simulink library "library_ALICAT_PRESSURE_RW"  (R2024b)
settings: Solver=VariableStepAuto  StartTime=0.0  StopTime=10.0  RelTol=1e-3
undefined symbols (not defined in the file): Controller
settings Model: Creator=GavinWilliamson  LastModifiedBy=GavinWilliamson

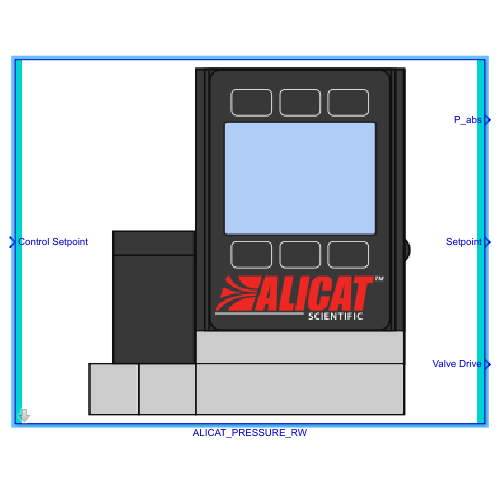
[thumbnail: Simulink's stored preview of the top-level diagram]
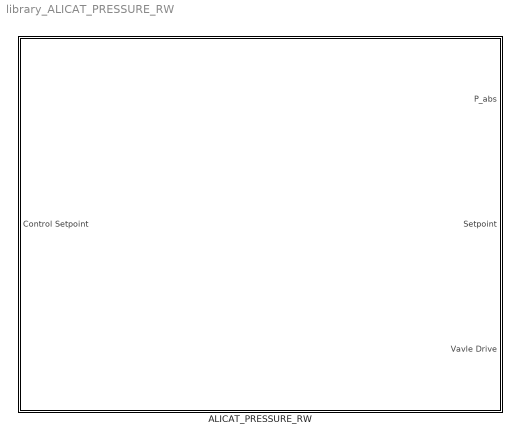
== system library_ALICAT_PRESSURE_RW ==
  ALICAT_PRESSURE_RW : Subsystem  mask{Port="COM4", Device_Name='A', dv_typ=Controller, vlv_typ=on, vlvDR_sw=on, cntrl_sw=on, contrl_typ=Absolute Pressure}
      mask prompts: Device_Name "Device Identifier"; dv_typ "Device Type"; vlv_typ "Two Valve Controller"; vlvDR_sw "Enable Valve Drive Recording"; cntrl_sw "Enable ALICAT Controller"; contrl_typ "Setpoint Variable"
      mask help: Default Mask
      mask Help: web(which('help_ALICAT_PRESSURE_RW.html'), '-helpbrowser')
      mask TypeOptions Port:
      | Level-2 MATLAB
      | S-Function/Port
      mask TypeOptions Device_Name:
      | Level-2 MATLAB
      | S-Function/Device_Name
      mask TypeOptions dv_typ:
      | Level-2 MATLAB
      | S-Function/dv_typ
      mask TypeOptions vlv_typ:
      | Level-2 MATLAB
      | S-Function/vlv_typ
      mask TypeOptions vlvDR_sw:
      | Level-2 MATLAB
      | S-Function/vlvDR_sw
      mask TypeOptions cntrl_sw:
      | Level-2 MATLAB
      | S-Function/cntrl_sw
      mask TypeOptions contrl_typ:
      | Level-2 MATLAB
      | S-Function/contrl_typ
      mask DialogControl Container3 Prompt: General
      mask DialogControl DescGroupVar_copy Prompt: ALICAT_RW
      mask DialogControl DescTextVar_copy Prompt: Block controls and reads an ALICAT pressure device over serial communication. Labels on the ports on the block will disappear if there are not valid for the configuration selected. To see all port labels you can look under the mask of this block.
      mask DialogControl Container10 Prompt: Communication Parameters
      mask DialogControl Container21 Prompt: Device Information
      mask DialogControl Container11 Prompt: Data Logging Options
      mask DialogControl Container12 Prompt: Control Options
      mask DialogControl Container5 Prompt: Instructions
      mask DialogControl Container6 Prompt: Inputs
      mask DialogControl Control2 Prompt: Control Setpoint: The setpoint that you want to write to the device if control mode is enabled. If control mode is disabled this input will no do anything.
      mask DialogControl Container7 Prompt: Register Parameters
      mask DialogControl Container18 Prompt: Communication Parameters
      mask DialogControl Control16 Prompt: Port: Communication port that ALICAT is connected to [string]
      mask DialogControl Control14 Prompt: Device Identifier: Unit ID of ALICAT [char]
      mask DialogControl Container13 Prompt: Device Information
      mask DialogControl Control7 Prompt: Device Type: Select whether the ALICAT that is connected to the COM Port is a controller or meter. This is important to ensure invalid commands are not sent to the device, and to ensure that the outputted data is in the expected format.
      mask DialogControl Control12 Prompt: Two Valve Controller: Select this option if you controller has two control valves
      mask DialogControl Container14 Prompt: Data Logging Options
      mask DialogControl Control8 Prompt: Enable Valve Drive Recording: This will set the valve drive position to be outputted by an ALICAT controller and will also set the value to display on the screen.
      mask DialogControl Container15 Prompt: Control Options
      mask DialogControl Control9 Prompt: Enable ALICAT Controller: This allows an ALICAT controller to be controlled through Simulink. If unchecked, Simulink will just configure the data logging option parameters and read the device outputs.
      mask DialogControl Container16 Prompt: Setpoint Variable
      mask DialogControl Control10 Prompt: If set to "Valve Drive", "Control Setpoint" should be set to the percentage open on the range of 0-100. Where 0 corresponds to closed and 100 corresponds to fully open.  If you have a two valve device the range 0-100 controls the left valve and  0 to -100 controls the right valve.
      mask Display:
      | image('AlicatMFCIcon.png', [0,0,0,0,100,100]);
      | 
      | %input ports
      | if strcmp(get_param(gcb,'cntrl_sw'),'on')
      |     port_label('input', 1, 'Control Setpoint');
      | end
      | 
      | %output ports
      | port_label('output', 1, 'P_abs');
      | if strcmp(get_param(gcb,'dv_typ'),'Controller')
      |     port_label('output', 2, 'Setpoint');
      | end
      | if strcmp(get_param(gcb,'vlvDr_sw'),'on')
      |     port_label('output', 3, 'Valve Drive');
      | end

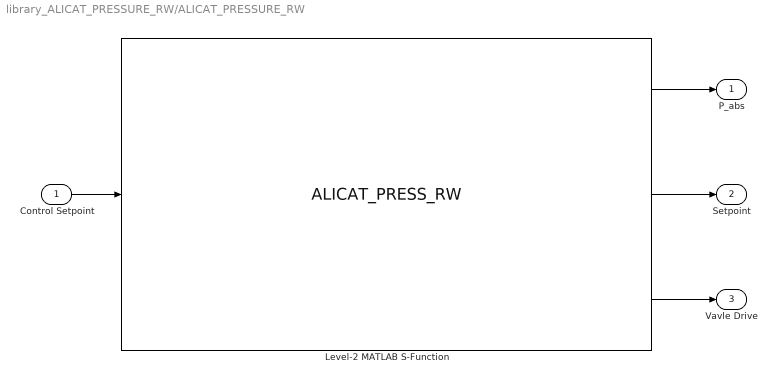
== system library_ALICAT_PRESSURE_RW/ALICAT_PRESSURE_RW ==
  Control Setpoint : Inport
  Level-2 MATLAB S-Function : M-S-Function  FunctionName=ALICAT_PRESS_RW  Parameters=Port, Device_Name, contrl_typ, cntrl_sw, dv_typ,vlvDR_sw,vlv_typ  mask{Port=Port, Device_Name=Device_Name, vlvDR_sw=on, cntrl_sw=on, contrl_typ=Absolute Pressure, dv_typ=Controller, vlv_typ=on}
      mask prompts: Device_Name "Device Identifier"; vlvDR_sw "Enable Valve Drive Recording"; cntrl_sw "Enable ALICAT Controller"; contrl_typ "Setpoint Variable"; dv_typ "Device Type"; vlv_typ "Two Valve Controller"
      mask TypeOptions contrl_typ: Absolute Pressure | Valve Drive
      mask TypeOptions dv_typ: Controller | Meter
      mask DialogControl DescGroupVar Prompt: ALICAT_RW
      mask DialogControl DescTextVar Prompt: *See mask of subsystem
      mask DialogControl Container4 Prompt: Connection Parameters
      mask DialogControl Container7 Prompt: Device Information
      mask DialogControl Container5 Prompt: Data Logging Options
      mask DialogControl Container6 Prompt: Control Options
      mask Display:
      | image('AlicatMFCIcon.png');
      | 
      | 
      | 
      | port_label('input', 1, 'Control Setpoint');
      | 
      | port_label('output', 1, 'P_abs');
      | port_label('output', 2, 'Setpoint');
      | port_label('output', 3, 'Valve Drive');
  P_abs : Outport
  Setpoint : Outport  Port=2
  Vavle Drive : Outport  Port=3
  wires:
  Control Setpoint/1 -> Level-2 MATLAB S-Function/1
  Level-2 MATLAB S-Function/1 -> P_abs/1
  Level-2 MATLAB S-Function/2 -> Setpoint/1
  Level-2 MATLAB S-Function/3 -> Vavle Drive/1
